simulink model "AFS"  (R2025b)
settings: Solver=VariableStepAuto  StartTime=0.0  StopTime=10.0  RelTol=1e-3
undefined symbols (not defined in the file): afs, dspblkCoreblockFVToolHelper, gcbh, solveAFSMPCOnline
settings Model: Creator=jaiden  LastModifiedBy=r3anjum

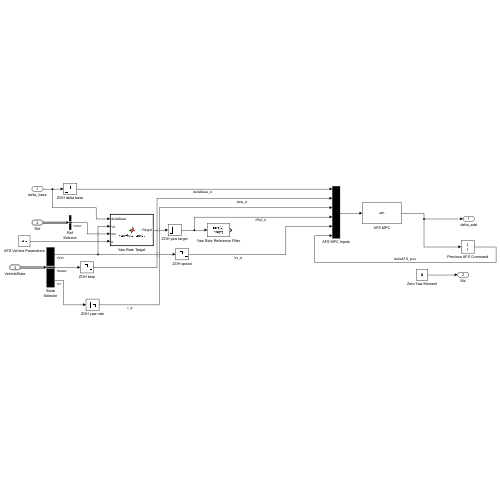
[thumbnail: Simulink's stored preview of the top-level diagram]
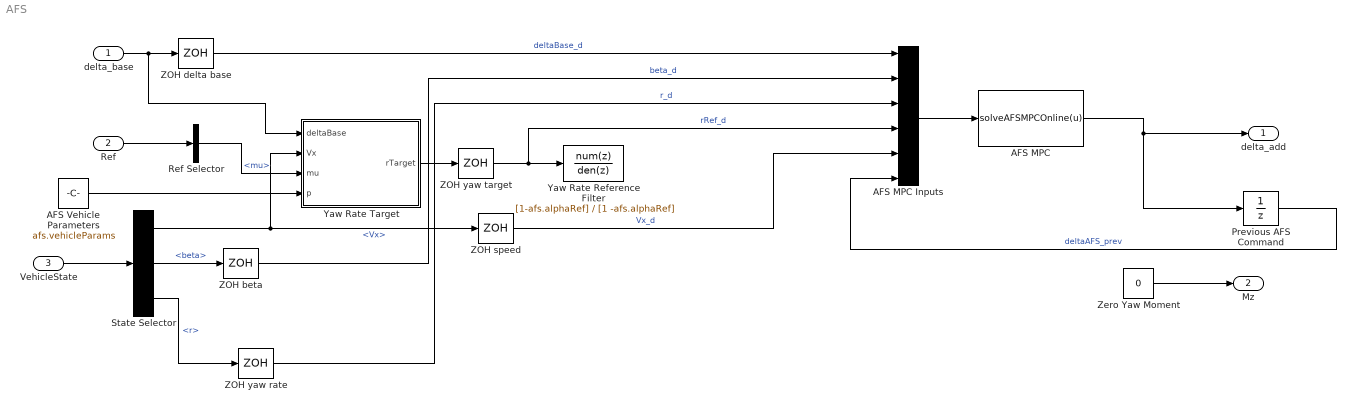
== system AFS ==
  delta_base : Inport
  Ref : Inport  Port=2  OutDataTypeStr=Bus: ReferenceBus
  VehicleState : Inport  Port=3  OutDataTypeStr=Bus: VehicleStateBus
  AFS MPC : MATLABFcn  MATLABFcn=solveAFSMPCOnline(u)  OutputDimensions=1  OutputSignalType=real
  AFS MPC Inputs : Mux  Inputs=6
  AFS Vehicle Parameters : Constant  Value=afs.vehicleParams
  Previous AFS Command : UnitDelay  SampleTime=afs.Ts  HasFrameUpgradeWarning=on
  Ref Selector : BusSelector  OutputSignals=mu
  State Selector : BusSelector  OutputSignals=Vx,beta,r
  Yaw Rate Reference Filter : DiscreteTransferFcn  LoadFcn=dspblkCoreblockFVToolHelper(gcbh,'load');  Numerator=[1-afs.alphaRef]  Denominator=[1 -afs.alphaRef]
      settings: CopyFcn=dspblkCoreblockFVToolHelper(gcbh,'copy');  DeleteFcn=dspblkCoreblockFVToolHelper(gcbh,'close');  ModelCloseFcn=dspblkCoreblockFVToolHelper(gcbh,'close');  PreSaveFcn=dspblkCoreblockFVToolHelper(gcbh,'presave');  PostSaveFcn=dspblkCoreblockFVToolHelper(gcbh,'postsave');  CloseFcn=dspblkCoreblockFVToolHelper(gcbh,'close');
  Yaw Rate Target : MATLAB Function  TreatAsAtomicUnit=on
  ZOH beta : ZeroOrderHold  SampleTime=afs.Ts
  ZOH delta base : ZeroOrderHold  SampleTime=afs.Ts
  ZOH speed : ZeroOrderHold  SampleTime=afs.Ts
  ZOH yaw rate : ZeroOrderHold  SampleTime=afs.Ts
  ZOH yaw target : ZeroOrderHold  SampleTime=afs.Ts
  Zero Yaw Moment : Constant  Value=0
  delta_add : Outport
  Mz : Outport  Port=2
  wires:
  Ref/1 -> Ref Selector/1
  VehicleState/1 -> State Selector/1
  State Selector/1 -> ZOH speed/1, Yaw Rate Target/2(Vx)  "<Vx>"
  Ref Selector/1 -> Yaw Rate Target/3(mu)  "<mu>"
  Yaw Rate Target/1(rTarget) -> ZOH yaw target/1
  ZOH yaw target/1 -> AFS MPC Inputs/4, Yaw Rate Reference Filter/1  "rRef_d"
  delta_base/1 -> Yaw Rate Target/1(deltaBase), ZOH delta base/1
  State Selector/2 -> ZOH beta/1  "<beta>"
  State Selector/3 -> ZOH yaw rate/1  "<r>"
  ZOH delta base/1 -> AFS MPC Inputs/1  "deltaBase_d"
  ZOH beta/1 -> AFS MPC Inputs/2  "beta_d"
  ZOH yaw rate/1 -> AFS MPC Inputs/3  "r_d"
  ZOH speed/1 -> AFS MPC Inputs/5  "Vx_d"
  Previous AFS Command/1 -> AFS MPC Inputs/6  "deltaAFS_prev"
  AFS MPC Inputs/1 -> AFS MPC/1
  Zero Yaw Moment/1 -> Mz/1
  AFS MPC/1 -> Previous AFS Command/1, delta_add/1
  AFS Vehicle Parameters/1 -> Yaw Rate Target/4(p)

== matlab function AFS/Yaw Rate Target ==
  data: deltaBase input; rTarget output; Vx input; mu input; p input
function rTarget = yawRateTarget(deltaBase, Vx, mu, p)
%#codegen
%
% Steering-based desired yaw rate for AFS.
%
% Inputs:
%   deltaBase : baseline road-wheel steering angle [rad]
%   Vx        : longitudinal speed [m/s]
%   mu        : road-friction coefficient
%   p         : [m; Iz; a; b; Caf; Car]
%
% Output:
%   rTarget   : desired yaw rate [rad/s]

g = 9.81;

m   = p(1);
a   = p(3);
b   = p(4);
Caf = p(5);
Car = p(6);

Vsafe = max(abs(Vx), 0.5);
L = a + b;

% Linear bicycle-model understeer coefficient.
Ku = (m/L)*(b/Caf - a/Car);

% Steady-state yaw-rate gain:
%
%   r_ss/delta = Vx/(L + Ku*Vx^2)
%
denominator = L + Ku*Vsafe^2;

% Numerical protection.
if abs(denominator) < 1e-6
    if denominator >= 0
        denominator = 1e-6;
    else
        denominator = -1e-6;
    end
end

rNominal = (Vsafe/denominator)*deltaBase;

% Friction-based yaw-rate limit.
rLimit = max(mu, 0)*g/Vsafe;

rTarget = min(max(rNominal, -rLimit), rLimit);

end
